simulink model "gpio_input_interrupt_am261"  (R2024b)
settings: Solver=FixedStepAuto  StartTime=0.0  StopTime=10.0  RelTol=1e-3
libraries: peripheral_library_blocks_am261x x3, HWI_lib x1
settings Model: Creator=a0499511  LastModifiedBy=a0499511
settings OptimizationCC: DefaultParameterBehavior=Inlined  EnhancedBackFolding=on  PassReuseOutputArgsAs=Individual arguments  ZeroExternalMemoryAtStartup=off  ZeroInternalMemoryAtStartup=off  MaxStackSize=64  OptimizeBlockOrder=speed  DifferentSizesBufferReuse=on  OptimizationCustomize=off  EfficientTunableParamExpr=on
settings DebuggingCC: ParameterTunabilityLossMsg=error
settings HardwareCC: ProdBitPerPointer=32  ProdBitPerSizeT=32  ProdBitPerPtrDiffT=32  ProdLargestAtomicInteger=Long  ProdLargestAtomicFloat=Double  ProdWordSize=32  ProdHWDeviceType=ARM Compatible->ARM Cortex
settings SFSimCC: MATLABDynamicMemAlloc=off
settings RTWCC: Description=Embedded Coder  SystemTargetFile=ert.tlc  HardwareBoard=AM261X LP  TemplateMakefile=ert_default_tmf  Toolchain=TI ARM Clang Compiler AM261x | gmake
settings CodeAppCC: ForceParamTrailComments=on  IgnoreCustomStorageClasses=off  OperatorAnnotations=on  SimulinkDataObjDesc=on  SFDataObjDesc=on  InsertBlockDesc=on
settings ERTTargetCC: SupportVariableSizeSignals=on

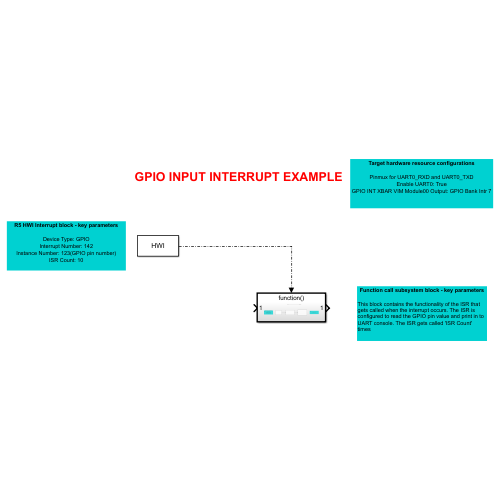
[thumbnail: Simulink's stored preview of the top-level diagram]
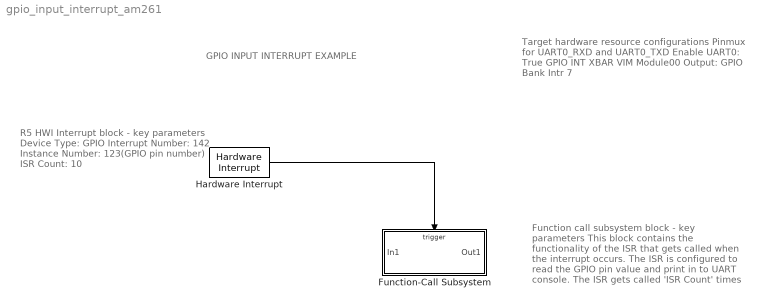
== system gpio_input_interrupt_am261 ==
  note: R5 HWI Interrupt block - key parameters
      |
      | Device Type: GPIO
      | Interrupt Number: 142
      | Instance Number: 123(GPIO pin number)
      | ISR Count: 10
  note: Function call subsystem block - key parameters
      |
      | This block contains the functionality of the ISR that gets called when the interrupt occurs. The ISR is configured to read the GPIO pin value and print in to UART console. The ISR gets called 'ISR Count' times
  note: GPIO INPUT INTERRUPT EXAMPLE
  note: Target hardware resource configurations
      |
      | Pinmux for UART0_RXD and UART0_TXD
      | Enable UART0: True
      | GPIO INT XBAR VIM Module00 Output: GPIO Bank Intr 7
  Function-Call Subsystem : Subsystem  TreatAsAtomicUnit=on
  Hardware Interrupt : HWI_lib/Hardware Interrupt  INTERRUPT_TYPE=GPIO  ISR_NUMBER=164  INSTANCE_NUMBER=124  SHOW_INPUTPORT=off
      settings: SourceProductName=Embedded Coder Support Package for AM263x - HWI Block
  wires:
  Hardware Interrupt/1 -> Function-Call Subsystem/Trigger

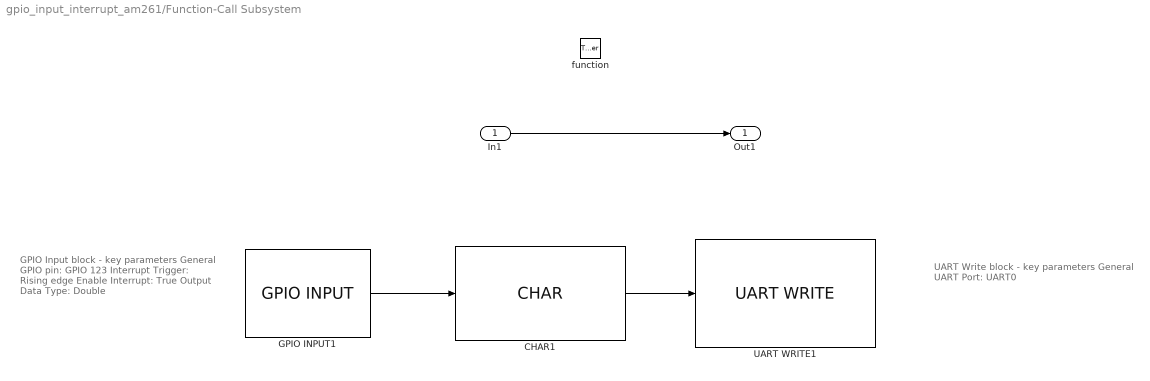
== system gpio_input_interrupt_am261/Function-Call Subsystem ==
  note: UART Write block - key parameters
      |
      | General
      | UART Port: UART0
  note: GPIO Input block - key parameters
      |
      | General
      | GPIO pin: GPIO 123
      | Interrupt Trigger: Rising edge
      | Enable Interrupt: True
      | Output Data Type: Double
  In1 : Inport
  function : TriggerPort  TriggerType=function-call  VariantControl=(inherit)
  CHAR1 : peripheral_library_blocks_am261x/CHAR
  GPIO INPUT1 : peripheral_library_blocks_am261x/GPIO INPUT  GPIO_Pin=GPIO124  Trigger_Type=Rising Edge  GPIOEnableInterrupt=on  Output_DataType=Double  SampleTime=-1
  UART WRITE1 : peripheral_library_blocks_am261x/UART WRITE  UARTPort=UART0
  Out1 : Outport
  wires:
  In1/1 -> Out1/1
  GPIO INPUT1/1 -> CHAR1/1
  CHAR1/1 -> UART WRITE1/1
